simulink model "CL_PC"  (R2022b)
settings: Solver=VariableStepAuto  StartTime=0.0  StopTime=10.0  RelTol=1e-3
settings Model: Creator=marcu  LastModifiedBy=marcu
settings ConfigComp: PLC_TargetIDE=codesys23  PLC_MultiTBSigbuilderTimeRange=off  PLC_FoldFBCallOutputVar=off  PLC_InlineEnumCastFunction=off

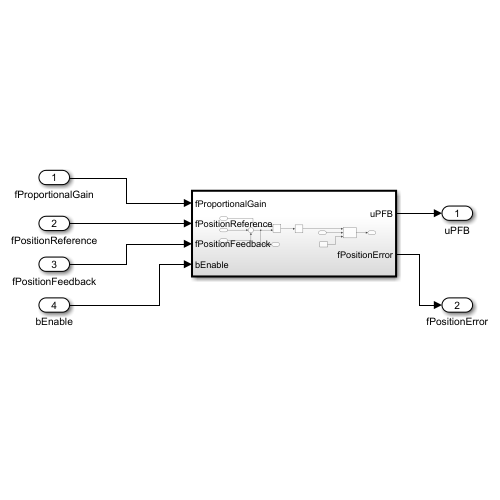
[thumbnail: Simulink's stored preview of the top-level diagram]
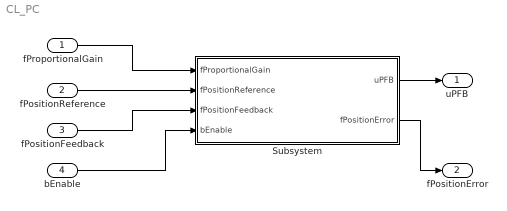
== system CL_PC ==
  fProportionalGain : Inport
  fPositionReference : Inport  Port=2
  fPositionFeedback : Inport  Port=3
  bEnable : Inport  Port=4
  Subsystem : Subsystem  TreatAsAtomicUnit=on
  uPFB : Outport
  fPositionError : Outport  Port=2
  wires:
  fProportionalGain/1 -> Subsystem/1(fProportionalGain)
  fPositionReference/1 -> Subsystem/2(fPositionReference)
  fPositionFeedback/1 -> Subsystem/3(fPositionFeedback)
  bEnable/1 -> Subsystem/4(bEnable)
  Subsystem/1(uPFB) -> uPFB/1
  Subsystem/2(fPositionError) -> fPositionError/1

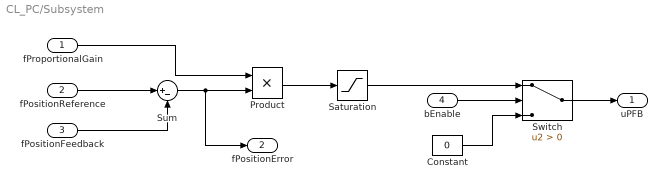
== system CL_PC/Subsystem ==
  fProportionalGain : Inport
  fPositionReference : Inport  Port=2
  fPositionFeedback : Inport  Port=3
  bEnable : Inport  Port=4
  Constant : Constant  Value=0
  Product : Product
  Saturation : Saturate
  Sum : Sum  Inputs=|+-
  Switch : Switch  Criteria=u2 > Threshold  SaturateOnIntegerOverflow=off  InputSameDT=off
  uPFB : Outport
  fPositionError : Outport  Port=2
  wires:
  Product/1 -> Saturation/1
  fProportionalGain/1 -> Product/1
  Sum/1 -> fPositionError/1, Product/2
  Constant/1 -> Switch/3
  Switch/1 -> uPFB/1
  fPositionReference/1 -> Sum/1
  fPositionFeedback/1 -> Sum/2
  Saturation/1 -> Switch/1
  bEnable/1 -> Switch/2
